simulink model "Filter_testaus_uusi"  (R2017b)
settings: Solver=FixedStepDiscrete  StartTime=0.0  StopTime=10  FixedStep=1/44100  RelTol=1e-3
(part 2 of 4)

== system Filter_testaus_uusi/Highpass/HighpassH/Resonator100 ==
  In1 : Inport
  Constant : Constant  Value=0i
  Delay : Delay  DelayLength=1
  Gain : Gain  Gain=-0.93539-0.3536i
  GainH : Gain  Gain=-0.16604+0.98612i
  Real-Imag to Complex : RealImagToComplex
  Sum1 : Sum  Inputs=|++
  Out1 : Outport
  wires:
  Constant/1 -> Real-Imag to Complex/2
  Real-Imag to Complex/1 -> Sum1/1
  In1/1 -> Real-Imag to Complex/1
  GainH/1 -> Out1/1
  Gain/1 -> Sum1/2
  Delay/1 -> Gain/1
  Sum1/1 -> Delay/1, GainH/1

== system Filter_testaus_uusi/Highpass/HighpassH/Resonator101 ==
  In1 : Inport
  Constant : Constant  Value=0i
  Delay : Delay  DelayLength=1
  Gain : Gain  Gain=-0.9252-0.37947i
  GainH : Gain  Gain=0.17973-0.98372i
  Real-Imag to Complex : RealImagToComplex
  Sum1 : Sum  Inputs=|++
  Out1 : Outport
  wires:
  Constant/1 -> Real-Imag to Complex/2
  Real-Imag to Complex/1 -> Sum1/1
  In1/1 -> Real-Imag to Complex/1
  GainH/1 -> Out1/1
  Gain/1 -> Sum1/2
  Delay/1 -> Gain/1
  Sum1/1 -> Delay/1, GainH/1

== system Filter_testaus_uusi/Highpass/HighpassH/Resonator102 ==
  In1 : Inport
  Constant : Constant  Value=0i
  Delay : Delay  DelayLength=1
  Gain : Gain  Gain=-0.9143-0.40504i
  GainH : Gain  Gain=-0.19339+0.98112i
  Real-Imag to Complex : RealImagToComplex
  Sum1 : Sum  Inputs=|++
  Out1 : Outport
  wires:
  Constant/1 -> Real-Imag to Complex/2
  Real-Imag to Complex/1 -> Sum1/1
  In1/1 -> Real-Imag to Complex/1
  GainH/1 -> Out1/1
  Gain/1 -> Sum1/2
  Delay/1 -> Gain/1
  Sum1/1 -> Delay/1, GainH/1

== system Filter_testaus_uusi/Highpass/HighpassH/Resonator103 ==
  In1 : Inport
  Constant : Constant  Value=0i
  Delay : Delay  DelayLength=1
  Gain : Gain  Gain=-0.90269-0.4303i
  GainH : Gain  Gain=0.20701-0.97834i
  Real-Imag to Complex : RealImagToComplex
  Sum1 : Sum  Inputs=|++
  Out1 : Outport
  wires:
  Constant/1 -> Real-Imag to Complex/2
  Real-Imag to Complex/1 -> Sum1/1
  In1/1 -> Real-Imag to Complex/1
  GainH/1 -> Out1/1
  Gain/1 -> Sum1/2
  Delay/1 -> Gain/1
  Sum1/1 -> Delay/1, GainH/1

== system Filter_testaus_uusi/Highpass/HighpassH/Resonator104 ==
  In1 : Inport
  Constant : Constant  Value=0i
  Delay : Delay  DelayLength=1
  Gain : Gain  Gain=-0.89037-0.45523i
  GainH : Gain  Gain=-0.22058+0.97537i
  Real-Imag to Complex : RealImagToComplex
  Sum1 : Sum  Inputs=|++
  Out1 : Outport
  wires:
  Constant/1 -> Real-Imag to Complex/2
  Real-Imag to Complex/1 -> Sum1/1
  In1/1 -> Real-Imag to Complex/1
  GainH/1 -> Out1/1
  Gain/1 -> Sum1/2
  Delay/1 -> Gain/1
  Sum1/1 -> Delay/1, GainH/1

== system Filter_testaus_uusi/Highpass/HighpassH/Resonator105 ==
  In1 : Inport
  Constant : Constant  Value=0i
  Delay : Delay  DelayLength=1
  Gain : Gain  Gain=-0.87738-0.4798i
  GainH : Gain  Gain=0.23412-0.97221i
  Real-Imag to Complex : RealImagToComplex
  Sum1 : Sum  Inputs=|++
  Out1 : Outport
  wires:
  Constant/1 -> Real-Imag to Complex/2
  Real-Imag to Complex/1 -> Sum1/1
  In1/1 -> Real-Imag to Complex/1
  GainH/1 -> Out1/1
  Gain/1 -> Sum1/2
  Delay/1 -> Gain/1
  Sum1/1 -> Delay/1, GainH/1

== system Filter_testaus_uusi/Highpass/HighpassH/Resonator106 ==
  In1 : Inport
  Constant : Constant  Value=0i
  Delay : Delay  DelayLength=1
  Gain : Gain  Gain=-0.8637-0.50401i
  GainH : Gain  Gain=-0.24761+0.96886i
  Real-Imag to Complex : RealImagToComplex
  Sum1 : Sum  Inputs=|++
  Out1 : Outport
  wires:
  Constant/1 -> Real-Imag to Complex/2
  Real-Imag to Complex/1 -> Sum1/1
  In1/1 -> Real-Imag to Complex/1
  GainH/1 -> Out1/1
  Gain/1 -> Sum1/2
  Delay/1 -> Gain/1
  Sum1/1 -> Delay/1, GainH/1

== system Filter_testaus_uusi/Highpass/HighpassH/Resonator107 ==
  In1 : Inport
  Constant : Constant  Value=0i
  Delay : Delay  DelayLength=1
  Gain : Gain  Gain=-0.84936-0.52782i
  GainH : Gain  Gain=0.26106-0.96532i
  Real-Imag to Complex : RealImagToComplex
  Sum1 : Sum  Inputs=|++
  Out1 : Outport
  wires:
  Constant/1 -> Real-Imag to Complex/2
  Real-Imag to Complex/1 -> Sum1/1
  In1/1 -> Real-Imag to Complex/1
  GainH/1 -> Out1/1
  Gain/1 -> Sum1/2
  Delay/1 -> Gain/1
  Sum1/1 -> Delay/1, GainH/1

== system Filter_testaus_uusi/Highpass/HighpassH/Resonator108 ==
  In1 : Inport
  Constant : Constant  Value=0i
  Delay : Delay  DelayLength=1
  Gain : Gain  Gain=-0.83435-0.55123i
  GainH : Gain  Gain=-0.27445+0.9616i
  Real-Imag to Complex : RealImagToComplex
  Sum1 : Sum  Inputs=|++
  Out1 : Outport
  wires:
  Constant/1 -> Real-Imag to Complex/2
  Real-Imag to Complex/1 -> Sum1/1
  In1/1 -> Real-Imag to Complex/1
  GainH/1 -> Out1/1
  Gain/1 -> Sum1/2
  Delay/1 -> Gain/1
  Sum1/1 -> Delay/1, GainH/1

== system Filter_testaus_uusi/Highpass/HighpassH/Resonator109 ==
  In1 : Inport
  Constant : Constant  Value=0i
  Delay : Delay  DelayLength=1
  Gain : Gain  Gain=-0.81871-0.57421i
  GainH : Gain  Gain=0.28779-0.95769i
  Real-Imag to Complex : RealImagToComplex
  Sum1 : Sum  Inputs=|++
  Out1 : Outport
  wires:
  Constant/1 -> Real-Imag to Complex/2
  Real-Imag to Complex/1 -> Sum1/1
  In1/1 -> Real-Imag to Complex/1
  GainH/1 -> Out1/1
  Gain/1 -> Sum1/2
  Delay/1 -> Gain/1
  Sum1/1 -> Delay/1, GainH/1

== system Filter_testaus_uusi/Highpass/HighpassH/Resonator11 ==
  In1 : Inport
  Constant : Constant  Value=0i
  Delay : Delay  DelayLength=1
  Gain : Gain  Gain=0.51596+0.85661i
  GainH : Gain  Gain=0.87738+0.4798i
  Real-Imag to Complex : RealImagToComplex
  Sum1 : Sum  Inputs=|++
  Out1 : Outport
  wires:
  Constant/1 -> Real-Imag to Complex/2
  Real-Imag to Complex/1 -> Sum1/1
  In1/1 -> Real-Imag to Complex/1
  GainH/1 -> Out1/1
  Gain/1 -> Sum1/2
  Delay/1 -> Gain/1
  Sum1/1 -> Delay/1, GainH/1

== system Filter_testaus_uusi/Highpass/HighpassH/Resonator110 ==
  In1 : Inport
  Constant : Constant  Value=0i
  Delay : Delay  DelayLength=1
  Gain : Gain  Gain=-0.80243-0.59675i
  GainH : Gain  Gain=-0.30107+0.9536i
  Real-Imag to Complex : RealImagToComplex
  Sum1 : Sum  Inputs=|++
  Out1 : Outport
  wires:
  Constant/1 -> Real-Imag to Complex/2
  Real-Imag to Complex/1 -> Sum1/1
  In1/1 -> Real-Imag to Complex/1
  GainH/1 -> Out1/1
  Gain/1 -> Sum1/2
  Delay/1 -> Gain/1
  Sum1/1 -> Delay/1, GainH/1

== system Filter_testaus_uusi/Highpass/HighpassH/Resonator111 ==
  In1 : Inport
  Constant : Constant  Value=0i
  Delay : Delay  DelayLength=1
  Gain : Gain  Gain=-0.78553-0.61882i
  GainH : Gain  Gain=0.3143-0.94932i
  Real-Imag to Complex : RealImagToComplex
  Sum1 : Sum  Inputs=|++
  Out1 : Outport
  wires:
  Constant/1 -> Real-Imag to Complex/2
  Real-Imag to Complex/1 -> Sum1/1
  In1/1 -> Real-Imag to Complex/1
  GainH/1 -> Out1/1
  Gain/1 -> Sum1/2
  Delay/1 -> Gain/1
  Sum1/1 -> Delay/1, GainH/1

== system Filter_testaus_uusi/Highpass/HighpassH/Resonator112 ==
  In1 : Inport
  Constant : Constant  Value=0i
  Delay : Delay  DelayLength=1
  Gain : Gain  Gain=-0.76803-0.64042i
  GainH : Gain  Gain=-0.32747+0.94486i
  Real-Imag to Complex : RealImagToComplex
  Sum1 : Sum  Inputs=|++
  Out1 : Outport
  wires:
  Constant/1 -> Real-Imag to Complex/2
  Real-Imag to Complex/1 -> Sum1/1
  In1/1 -> Real-Imag to Complex/1
  GainH/1 -> Out1/1
  Gain/1 -> Sum1/2
  Delay/1 -> Gain/1
  Sum1/1 -> Delay/1, GainH/1

== system Filter_testaus_uusi/Highpass/HighpassH/Resonator113 ==
  In1 : Inport
  Constant : Constant  Value=0i
  Delay : Delay  DelayLength=1
  Gain : Gain  Gain=-0.74993-0.66152i
  GainH : Gain  Gain=0.34057-0.94022i
  Real-Imag to Complex : RealImagToComplex
  Sum1 : Sum  Inputs=|++
  Out1 : Outport
  wires:
  Constant/1 -> Real-Imag to Complex/2
  Real-Imag to Complex/1 -> Sum1/1
  In1/1 -> Real-Imag to Complex/1
  GainH/1 -> Out1/1
  Gain/1 -> Sum1/2
  Delay/1 -> Gain/1
  Sum1/1 -> Delay/1, GainH/1

== system Filter_testaus_uusi/Highpass/HighpassH/Resonator114 ==
  In1 : Inport
  Constant : Constant  Value=0i
  Delay : Delay  DelayLength=1
  Gain : Gain  Gain=-0.73125-0.68211i
  GainH : Gain  Gain=-0.3536+0.93539i
  Real-Imag to Complex : RealImagToComplex
  Sum1 : Sum  Inputs=|++
  Out1 : Outport
  wires:
  Constant/1 -> Real-Imag to Complex/2
  Real-Imag to Complex/1 -> Sum1/1
  In1/1 -> Real-Imag to Complex/1
  GainH/1 -> Out1/1
  Gain/1 -> Sum1/2
  Delay/1 -> Gain/1
  Sum1/1 -> Delay/1, GainH/1

== system Filter_testaus_uusi/Highpass/HighpassH/Resonator115 ==
  In1 : Inport
  Constant : Constant  Value=0i
  Delay : Delay  DelayLength=1
  Gain : Gain  Gain=-0.712-0.70218i
  GainH : Gain  Gain=0.36657-0.93039i
  Real-Imag to Complex : RealImagToComplex
  Sum1 : Sum  Inputs=|++
  Out1 : Outport
  wires:
  Constant/1 -> Real-Imag to Complex/2
  Real-Imag to Complex/1 -> Sum1/1
  In1/1 -> Real-Imag to Complex/1
  GainH/1 -> Out1/1
  Gain/1 -> Sum1/2
  Delay/1 -> Gain/1
  Sum1/1 -> Delay/1, GainH/1

== system Filter_testaus_uusi/Highpass/HighpassH/Resonator116 ==
  In1 : Inport
  Constant : Constant  Value=0i
  Delay : Delay  DelayLength=1
  Gain : Gain  Gain=-0.69221-0.7217i
  GainH : Gain  Gain=-0.37947+0.9252i
  Real-Imag to Complex : RealImagToComplex
  Sum1 : Sum  Inputs=|++
  Out1 : Outport
  wires:
  Constant/1 -> Real-Imag to Complex/2
  Real-Imag to Complex/1 -> Sum1/1
  In1/1 -> Real-Imag to Complex/1
  GainH/1 -> Out1/1
  Gain/1 -> Sum1/2
  Delay/1 -> Gain/1
  Sum1/1 -> Delay/1, GainH/1

== system Filter_testaus_uusi/Highpass/HighpassH/Resonator117 ==
  In1 : Inport
  Constant : Constant  Value=0i
  Delay : Delay  DelayLength=1
  Gain : Gain  Gain=-0.67188-0.74066i
  GainH : Gain  Gain=0.39229-0.91984i
  Real-Imag to Complex : RealImagToComplex
  Sum1 : Sum  Inputs=|++
  Out1 : Outport
  wires:
  Constant/1 -> Real-Imag to Complex/2
  Real-Imag to Complex/1 -> Sum1/1
  In1/1 -> Real-Imag to Complex/1
  GainH/1 -> Out1/1
  Gain/1 -> Sum1/2
  Delay/1 -> Gain/1
  Sum1/1 -> Delay/1, GainH/1

== system Filter_testaus_uusi/Highpass/HighpassH/Resonator118 ==
  In1 : Inport
  Constant : Constant  Value=0i
  Delay : Delay  DelayLength=1
  Gain : Gain  Gain=-0.65103-0.75905i
  GainH : Gain  Gain=-0.40504+0.9143i
  Real-Imag to Complex : RealImagToComplex
  Sum1 : Sum  Inputs=|++
  Out1 : Outport
  wires:
  Constant/1 -> Real-Imag to Complex/2
  Real-Imag to Complex/1 -> Sum1/1
  In1/1 -> Real-Imag to Complex/1
  GainH/1 -> Out1/1
  Gain/1 -> Sum1/2
  Delay/1 -> Gain/1
  Sum1/1 -> Delay/1, GainH/1

== system Filter_testaus_uusi/Highpass/HighpassH/Resonator119 ==
  In1 : Inport
  Constant : Constant  Value=0i
  Delay : Delay  DelayLength=1
  Gain : Gain  Gain=-0.62968-0.77685i
  GainH : Gain  Gain=0.41771-0.90858i
  Real-Imag to Complex : RealImagToComplex
  Sum1 : Sum  Inputs=|++
  Out1 : Outport
  wires:
  Constant/1 -> Real-Imag to Complex/2
  Real-Imag to Complex/1 -> Sum1/1
  In1/1 -> Real-Imag to Complex/1
  GainH/1 -> Out1/1
  Gain/1 -> Sum1/2
  Delay/1 -> Gain/1
  Sum1/1 -> Delay/1, GainH/1

== system Filter_testaus_uusi/Highpass/HighpassH/Resonator12 ==
  In1 : Inport
  Constant : Constant  Value=0i
  Delay : Delay  DelayLength=1
  Gain : Gain  Gain=0.49195+0.87062i
  GainH : Gain  Gain=-0.87062-0.49195i
  Real-Imag to Complex : RealImagToComplex
  Sum1 : Sum  Inputs=|++
  Out1 : Outport
  wires:
  Constant/1 -> Real-Imag to Complex/2
  Real-Imag to Complex/1 -> Sum1/1
  In1/1 -> Real-Imag to Complex/1
  GainH/1 -> Out1/1
  Gain/1 -> Sum1/2
  Delay/1 -> Gain/1
  Sum1/1 -> Delay/1, GainH/1

== system Filter_testaus_uusi/Highpass/HighpassH/Resonator120 ==
  In1 : Inport
  Constant : Constant  Value=0i
  Delay : Delay  DelayLength=1
  Gain : Gain  Gain=-0.60784-0.79406i
  GainH : Gain  Gain=-0.4303+0.90269i
  Real-Imag to Complex : RealImagToComplex
  Sum1 : Sum  Inputs=|++
  Out1 : Outport
  wires:
  Constant/1 -> Real-Imag to Complex/2
  Real-Imag to Complex/1 -> Sum1/1
  In1/1 -> Real-Imag to Complex/1
  GainH/1 -> Out1/1
  Gain/1 -> Sum1/2
  Delay/1 -> Gain/1
  Sum1/1 -> Delay/1, GainH/1

== system Filter_testaus_uusi/Highpass/HighpassH/Resonator121 ==
  In1 : Inport
  Constant : Constant  Value=0i
  Delay : Delay  DelayLength=1
  Gain : Gain  Gain=-0.58553-0.81065i
  GainH : Gain  Gain=0.44281-0.89662i
  Real-Imag to Complex : RealImagToComplex
  Sum1 : Sum  Inputs=|++
  Out1 : Outport
  wires:
  Constant/1 -> Real-Imag to Complex/2
  Real-Imag to Complex/1 -> Sum1/1
  In1/1 -> Real-Imag to Complex/1
  GainH/1 -> Out1/1
  Gain/1 -> Sum1/2
  Delay/1 -> Gain/1
  Sum1/1 -> Delay/1, GainH/1

== system Filter_testaus_uusi/Highpass/HighpassH/Resonator122 ==
  In1 : Inport
  Constant : Constant  Value=0i
  Delay : Delay  DelayLength=1
  Gain : Gain  Gain=-0.56277-0.82661i
  GainH : Gain  Gain=-0.45523+0.89037i
  Real-Imag to Complex : RealImagToComplex
  Sum1 : Sum  Inputs=|++
  Out1 : Outport
  wires:
  Constant/1 -> Real-Imag to Complex/2
  Real-Imag to Complex/1 -> Sum1/1
  In1/1 -> Real-Imag to Complex/1
  GainH/1 -> Out1/1
  Gain/1 -> Sum1/2
  Delay/1 -> Gain/1
  Sum1/1 -> Delay/1, GainH/1

== system Filter_testaus_uusi/Highpass/HighpassH/Resonator123 ==
  In1 : Inport
  Constant : Constant  Value=0i
  Delay : Delay  DelayLength=1
  Gain : Gain  Gain=-0.53958-0.84194i
  GainH : Gain  Gain=0.46756-0.88396i
  Real-Imag to Complex : RealImagToComplex
  Sum1 : Sum  Inputs=|++
  Out1 : Outport
  wires:
  Constant/1 -> Real-Imag to Complex/2
  Real-Imag to Complex/1 -> Sum1/1
  In1/1 -> Real-Imag to Complex/1
  GainH/1 -> Out1/1
  Gain/1 -> Sum1/2
  Delay/1 -> Gain/1
  Sum1/1 -> Delay/1, GainH/1

== system Filter_testaus_uusi/Highpass/HighpassH/Resonator124 ==
  In1 : Inport
  Constant : Constant  Value=0i
  Delay : Delay  DelayLength=1
  Gain : Gain  Gain=-0.51596-0.85661i
  GainH : Gain  Gain=-0.4798+0.87738i
  Real-Imag to Complex : RealImagToComplex
  Sum1 : Sum  Inputs=|++
  Out1 : Outport
  wires:
  Constant/1 -> Real-Imag to Complex/2
  Real-Imag to Complex/1 -> Sum1/1
  In1/1 -> Real-Imag to Complex/1
  GainH/1 -> Out1/1
  Gain/1 -> Sum1/2
  Delay/1 -> Gain/1
  Sum1/1 -> Delay/1, GainH/1

== system Filter_testaus_uusi/Highpass/HighpassH/Resonator125 ==
  In1 : Inport
  Constant : Constant  Value=0i
  Delay : Delay  DelayLength=1
  Gain : Gain  Gain=-0.49195-0.87062i
  GainH : Gain  Gain=0.49195-0.87062i
  Real-Imag to Complex : RealImagToComplex
  Sum1 : Sum  Inputs=|++
  Out1 : Outport
  wires:
  Constant/1 -> Real-Imag to Complex/2
  Real-Imag to Complex/1 -> Sum1/1
  In1/1 -> Real-Imag to Complex/1
  GainH/1 -> Out1/1
  Gain/1 -> Sum1/2
  Delay/1 -> Gain/1
  Sum1/1 -> Delay/1, GainH/1

== system Filter_testaus_uusi/Highpass/HighpassH/Resonator126 ==
  In1 : Inport
  Constant : Constant  Value=0i
  Delay : Delay  DelayLength=1
  Gain : Gain  Gain=-0.46756-0.88396i
  GainH : Gain  Gain=-0.50401+0.8637i
  Real-Imag to Complex : RealImagToComplex
  Sum1 : Sum  Inputs=|++
  Out1 : Outport
  wires:
  Constant/1 -> Real-Imag to Complex/2
  Real-Imag to Complex/1 -> Sum1/1
  In1/1 -> Real-Imag to Complex/1
  GainH/1 -> Out1/1
  Gain/1 -> Sum1/2
  Delay/1 -> Gain/1
  Sum1/1 -> Delay/1, GainH/1

== system Filter_testaus_uusi/Highpass/HighpassH/Resonator127 ==
  In1 : Inport
  Constant : Constant  Value=0i
  Delay : Delay  DelayLength=1
  Gain : Gain  Gain=-0.44281-0.89662i
  GainH : Gain  Gain=0.51596-0.85661i
  Real-Imag to Complex : RealImagToComplex
  Sum1 : Sum  Inputs=|++
  Out1 : Outport
  wires:
  Constant/1 -> Real-Imag to Complex/2
  Real-Imag to Complex/1 -> Sum1/1
  In1/1 -> Real-Imag to Complex/1
  GainH/1 -> Out1/1
  Gain/1 -> Sum1/2
  Delay/1 -> Gain/1
  Sum1/1 -> Delay/1, GainH/1

== system Filter_testaus_uusi/Highpass/HighpassH/Resonator128 ==
  In1 : Inport
  Constant : Constant  Value=0i
  Delay : Delay  DelayLength=1
  Gain : Gain  Gain=-0.41771-0.90858i
  GainH : Gain  Gain=-0.52782+0.84936i
  Real-Imag to Complex : RealImagToComplex
  Sum1 : Sum  Inputs=|++
  Out1 : Outport
  wires:
  Constant/1 -> Real-Imag to Complex/2
  Real-Imag to Complex/1 -> Sum1/1
  In1/1 -> Real-Imag to Complex/1
  GainH/1 -> Out1/1
  Gain/1 -> Sum1/2
  Delay/1 -> Gain/1
  Sum1/1 -> Delay/1, GainH/1

== system Filter_testaus_uusi/Highpass/HighpassH/Resonator129 ==
  In1 : Inport
  Constant : Constant  Value=0i
  Delay : Delay  DelayLength=1
  Gain : Gain  Gain=-0.39229-0.91984i
  GainH : Gain  Gain=0.53958-0.84194i
  Real-Imag to Complex : RealImagToComplex
  Sum1 : Sum  Inputs=|++
  Out1 : Outport
  wires:
  Constant/1 -> Real-Imag to Complex/2
  Real-Imag to Complex/1 -> Sum1/1
  In1/1 -> Real-Imag to Complex/1
  GainH/1 -> Out1/1
  Gain/1 -> Sum1/2
  Delay/1 -> Gain/1
  Sum1/1 -> Delay/1, GainH/1

== system Filter_testaus_uusi/Highpass/HighpassH/Resonator13 ==
  In1 : Inport
  Constant : Constant  Value=0i
  Delay : Delay  DelayLength=1
  Gain : Gain  Gain=0.46756+0.88396i
  GainH : Gain  Gain=0.8637+0.50401i
  Real-Imag to Complex : RealImagToComplex
  Sum1 : Sum  Inputs=|++
  Out1 : Outport
  wires:
  Constant/1 -> Real-Imag to Complex/2
  Real-Imag to Complex/1 -> Sum1/1
  In1/1 -> Real-Imag to Complex/1
  GainH/1 -> Out1/1
  Gain/1 -> Sum1/2
  Delay/1 -> Gain/1
  Sum1/1 -> Delay/1, GainH/1

== system Filter_testaus_uusi/Highpass/HighpassH/Resonator130 ==
  In1 : Inport
  Constant : Constant  Value=0i
  Delay : Delay  DelayLength=1
  Gain : Gain  Gain=-0.36657-0.93039i
  GainH : Gain  Gain=-0.55123+0.83435i
  Real-Imag to Complex : RealImagToComplex
  Sum1 : Sum  Inputs=|++
  Out1 : Outport
  wires:
  Constant/1 -> Real-Imag to Complex/2
  Real-Imag to Complex/1 -> Sum1/1
  In1/1 -> Real-Imag to Complex/1
  GainH/1 -> Out1/1
  Gain/1 -> Sum1/2
  Delay/1 -> Gain/1
  Sum1/1 -> Delay/1, GainH/1

== system Filter_testaus_uusi/Highpass/HighpassH/Resonator131 ==
  In1 : Inport
  Constant : Constant  Value=0i
  Delay : Delay  DelayLength=1
  Gain : Gain  Gain=-0.34057-0.94022i
  GainH : Gain  Gain=0.56277-0.82661i
  Real-Imag to Complex : RealImagToComplex
  Sum1 : Sum  Inputs=|++
  Out1 : Outport
  wires:
  Constant/1 -> Real-Imag to Complex/2
  Real-Imag to Complex/1 -> Sum1/1
  In1/1 -> Real-Imag to Complex/1
  GainH/1 -> Out1/1
  Gain/1 -> Sum1/2
  Delay/1 -> Gain/1
  Sum1/1 -> Delay/1, GainH/1

== system Filter_testaus_uusi/Highpass/HighpassH/Resonator132 ==
  In1 : Inport
  Constant : Constant  Value=0i
  Delay : Delay  DelayLength=1
  Gain : Gain  Gain=-0.3143-0.94932i
  GainH : Gain  Gain=-0.57421+0.81871i
  Real-Imag to Complex : RealImagToComplex
  Sum1 : Sum  Inputs=|++
  Out1 : Outport
  wires:
  Constant/1 -> Real-Imag to Complex/2
  Real-Imag to Complex/1 -> Sum1/1
  In1/1 -> Real-Imag to Complex/1
  GainH/1 -> Out1/1
  Gain/1 -> Sum1/2
  Delay/1 -> Gain/1
  Sum1/1 -> Delay/1, GainH/1

== system Filter_testaus_uusi/Highpass/HighpassH/Resonator133 ==
  In1 : Inport
  Constant : Constant  Value=0i
  Delay : Delay  DelayLength=1
  Gain : Gain  Gain=-0.28779-0.95769i
  GainH : Gain  Gain=0.58553-0.81065i
  Real-Imag to Complex : RealImagToComplex
  Sum1 : Sum  Inputs=|++
  Out1 : Outport
  wires:
  Constant/1 -> Real-Imag to Complex/2
  Real-Imag to Complex/1 -> Sum1/1
  In1/1 -> Real-Imag to Complex/1
  GainH/1 -> Out1/1
  Gain/1 -> Sum1/2
  Delay/1 -> Gain/1
  Sum1/1 -> Delay/1, GainH/1

== system Filter_testaus_uusi/Highpass/HighpassH/Resonator134 ==
  In1 : Inport
  Constant : Constant  Value=0i
  Delay : Delay  DelayLength=1
  Gain : Gain  Gain=-0.26106-0.96532i
  GainH : Gain  Gain=-0.59675+0.80243i
  Real-Imag to Complex : RealImagToComplex
  Sum1 : Sum  Inputs=|++
  Out1 : Outport
  wires:
  Constant/1 -> Real-Imag to Complex/2
  Real-Imag to Complex/1 -> Sum1/1
  In1/1 -> Real-Imag to Complex/1
  GainH/1 -> Out1/1
  Gain/1 -> Sum1/2
  Delay/1 -> Gain/1
  Sum1/1 -> Delay/1, GainH/1

== system Filter_testaus_uusi/Highpass/HighpassH/Resonator135 ==
  In1 : Inport
  Constant : Constant  Value=0i
  Delay : Delay  DelayLength=1
  Gain : Gain  Gain=-0.23412-0.97221i
  GainH : Gain  Gain=0.60784-0.79406i
  Real-Imag to Complex : RealImagToComplex
  Sum1 : Sum  Inputs=|++
  Out1 : Outport
  wires:
  Constant/1 -> Real-Imag to Complex/2
  Real-Imag to Complex/1 -> Sum1/1
  In1/1 -> Real-Imag to Complex/1
  GainH/1 -> Out1/1
  Gain/1 -> Sum1/2
  Delay/1 -> Gain/1
  Sum1/1 -> Delay/1, GainH/1

== system Filter_testaus_uusi/Highpass/HighpassH/Resonator136 ==
  In1 : Inport
  Constant : Constant  Value=0i
  Delay : Delay  DelayLength=1
  Gain : Gain  Gain=-0.20701-0.97834i
  GainH : Gain  Gain=-0.61882+0.78553i
  Real-Imag to Complex : RealImagToComplex
  Sum1 : Sum  Inputs=|++
  Out1 : Outport
  wires:
  Constant/1 -> Real-Imag to Complex/2
  Real-Imag to Complex/1 -> Sum1/1
  In1/1 -> Real-Imag to Complex/1
  GainH/1 -> Out1/1
  Gain/1 -> Sum1/2
  Delay/1 -> Gain/1
  Sum1/1 -> Delay/1, GainH/1

== system Filter_testaus_uusi/Highpass/HighpassH/Resonator137 ==
  In1 : Inport
  Constant : Constant  Value=0i
  Delay : Delay  DelayLength=1
  Gain : Gain  Gain=-0.17973-0.98372i
  GainH : Gain  Gain=0.62968-0.77685i
  Real-Imag to Complex : RealImagToComplex
  Sum1 : Sum  Inputs=|++
  Out1 : Outport
  wires:
  Constant/1 -> Real-Imag to Complex/2
  Real-Imag to Complex/1 -> Sum1/1
  In1/1 -> Real-Imag to Complex/1
  GainH/1 -> Out1/1
  Gain/1 -> Sum1/2
  Delay/1 -> Gain/1
  Sum1/1 -> Delay/1, GainH/1

== system Filter_testaus_uusi/Highpass/HighpassH/Resonator138 ==
  In1 : Inport
  Constant : Constant  Value=0i
  Delay : Delay  DelayLength=1
  Gain : Gain  Gain=-0.15231-0.98833i
  GainH : Gain  Gain=-0.64042+0.76803i
  Real-Imag to Complex : RealImagToComplex
  Sum1 : Sum  Inputs=|++
  Out1 : Outport
  wires:
  Constant/1 -> Real-Imag to Complex/2
  Real-Imag to Complex/1 -> Sum1/1
  In1/1 -> Real-Imag to Complex/1
  GainH/1 -> Out1/1
  Gain/1 -> Sum1/2
  Delay/1 -> Gain/1
  Sum1/1 -> Delay/1, GainH/1

== system Filter_testaus_uusi/Highpass/HighpassH/Resonator139 ==
  In1 : Inport
  Constant : Constant  Value=0i
  Delay : Delay  DelayLength=1
  Gain : Gain  Gain=-0.12478-0.99218i
  GainH : Gain  Gain=0.65103-0.75905i
  Real-Imag to Complex : RealImagToComplex
  Sum1 : Sum  Inputs=|++
  Out1 : Outport
  wires:
  Constant/1 -> Real-Imag to Complex/2
  Real-Imag to Complex/1 -> Sum1/1
  In1/1 -> Real-Imag to Complex/1
  GainH/1 -> Out1/1
  Gain/1 -> Sum1/2
  Delay/1 -> Gain/1
  Sum1/1 -> Delay/1, GainH/1

== system Filter_testaus_uusi/Highpass/HighpassH/Resonator14 ==
  In1 : Inport
  Constant : Constant  Value=0i
  Delay : Delay  DelayLength=1
  Gain : Gain  Gain=0.44281+0.89662i
  GainH : Gain  Gain=-0.85661-0.51596i
  Real-Imag to Complex : RealImagToComplex
  Sum1 : Sum  Inputs=|++
  Out1 : Outport
  wires:
  Constant/1 -> Real-Imag to Complex/2
  Real-Imag to Complex/1 -> Sum1/1
  In1/1 -> Real-Imag to Complex/1
  GainH/1 -> Out1/1
  Gain/1 -> Sum1/2
  Delay/1 -> Gain/1
  Sum1/1 -> Delay/1, GainH/1

== system Filter_testaus_uusi/Highpass/HighpassH/Resonator140 ==
  In1 : Inport
  Constant : Constant  Value=0i
  Delay : Delay  DelayLength=1
  Gain : Gain  Gain=-0.097152-0.99527i
  GainH : Gain  Gain=-0.66152+0.74993i
  Real-Imag to Complex : RealImagToComplex
  Sum1 : Sum  Inputs=|++
  Out1 : Outport
  wires:
  Constant/1 -> Real-Imag to Complex/2
  Real-Imag to Complex/1 -> Sum1/1
  In1/1 -> Real-Imag to Complex/1
  GainH/1 -> Out1/1
  Gain/1 -> Sum1/2
  Delay/1 -> Gain/1
  Sum1/1 -> Delay/1, GainH/1

== system Filter_testaus_uusi/Highpass/HighpassH/Resonator141 ==
  In1 : Inport
  Constant : Constant  Value=0i
  Delay : Delay  DelayLength=1
  Gain : Gain  Gain=-0.069448-0.99759i
  GainH : Gain  Gain=0.67188-0.74066i
  Real-Imag to Complex : RealImagToComplex
  Sum1 : Sum  Inputs=|++
  Out1 : Outport
  wires:
  Constant/1 -> Real-Imag to Complex/2
  Real-Imag to Complex/1 -> Sum1/1
  In1/1 -> Real-Imag to Complex/1
  GainH/1 -> Out1/1
  Gain/1 -> Sum1/2
  Delay/1 -> Gain/1
  Sum1/1 -> Delay/1, GainH/1

== system Filter_testaus_uusi/Highpass/HighpassH/Resonator142 ==
  In1 : Inport
  Constant : Constant  Value=0i
  Delay : Delay  DelayLength=1
  Gain : Gain  Gain=-0.04169-0.99913i
  GainH : Gain  Gain=-0.68211+0.73125i
  Real-Imag to Complex : RealImagToComplex
  Sum1 : Sum  Inputs=|++
  Out1 : Outport
  wires:
  Constant/1 -> Real-Imag to Complex/2
  Real-Imag to Complex/1 -> Sum1/1
  In1/1 -> Real-Imag to Complex/1
  GainH/1 -> Out1/1
  Gain/1 -> Sum1/2
  Delay/1 -> Gain/1
  Sum1/1 -> Delay/1, GainH/1

== system Filter_testaus_uusi/Highpass/HighpassH/Resonator143 ==
  In1 : Inport
  Constant : Constant  Value=0i
  Delay : Delay  DelayLength=1
  Gain : Gain  Gain=-0.0139-0.9999i
  GainH : Gain  Gain=0.69221-0.7217i
  Real-Imag to Complex : RealImagToComplex
  Sum1 : Sum  Inputs=|++
  Out1 : Outport
  wires:
  Constant/1 -> Real-Imag to Complex/2
  Real-Imag to Complex/1 -> Sum1/1
  In1/1 -> Real-Imag to Complex/1
  GainH/1 -> Out1/1
  Gain/1 -> Sum1/2
  Delay/1 -> Gain/1
  Sum1/1 -> Delay/1, GainH/1

== system Filter_testaus_uusi/Highpass/HighpassH/Resonator144 ==
  In1 : Inport
  Constant : Constant  Value=0i
  Delay : Delay  DelayLength=1
  Gain : Gain  Gain=0.0139-0.9999i
  GainH : Gain  Gain=-0.70218+0.712i
  Real-Imag to Complex : RealImagToComplex
  Sum1 : Sum  Inputs=|++
  Out1 : Outport
  wires:
  Constant/1 -> Real-Imag to Complex/2
  Real-Imag to Complex/1 -> Sum1/1
  In1/1 -> Real-Imag to Complex/1
  GainH/1 -> Out1/1
  Gain/1 -> Sum1/2
  Delay/1 -> Gain/1
  Sum1/1 -> Delay/1, GainH/1

== system Filter_testaus_uusi/Highpass/HighpassH/Resonator145 ==
  In1 : Inport
  Constant : Constant  Value=0i
  Delay : Delay  DelayLength=1
  Gain : Gain  Gain=0.04169-0.99913i
  GainH : Gain  Gain=0.712-0.70218i
  Real-Imag to Complex : RealImagToComplex
  Sum1 : Sum  Inputs=|++
  Out1 : Outport
  wires:
  Constant/1 -> Real-Imag to Complex/2
  Real-Imag to Complex/1 -> Sum1/1
  In1/1 -> Real-Imag to Complex/1
  GainH/1 -> Out1/1
  Gain/1 -> Sum1/2
  Delay/1 -> Gain/1
  Sum1/1 -> Delay/1, GainH/1

== system Filter_testaus_uusi/Highpass/HighpassH/Resonator146 ==
  In1 : Inport
  Constant : Constant  Value=0i
  Delay : Delay  DelayLength=1
  Gain : Gain  Gain=0.069448-0.99759i
  GainH : Gain  Gain=-0.7217+0.69221i
  Real-Imag to Complex : RealImagToComplex
  Sum1 : Sum  Inputs=|++
  Out1 : Outport
  wires:
  Constant/1 -> Real-Imag to Complex/2
  Real-Imag to Complex/1 -> Sum1/1
  In1/1 -> Real-Imag to Complex/1
  GainH/1 -> Out1/1
  Gain/1 -> Sum1/2
  Delay/1 -> Gain/1
  Sum1/1 -> Delay/1, GainH/1

== system Filter_testaus_uusi/Highpass/HighpassH/Resonator147 ==
  In1 : Inport
  Constant : Constant  Value=0i
  Delay : Delay  DelayLength=1
  Gain : Gain  Gain=0.097152-0.99527i
  GainH : Gain  Gain=0.73125-0.68211i
  Real-Imag to Complex : RealImagToComplex
  Sum1 : Sum  Inputs=|++
  Out1 : Outport
  wires:
  Constant/1 -> Real-Imag to Complex/2
  Real-Imag to Complex/1 -> Sum1/1
  In1/1 -> Real-Imag to Complex/1
  GainH/1 -> Out1/1
  Gain/1 -> Sum1/2
  Delay/1 -> Gain/1
  Sum1/1 -> Delay/1, GainH/1

== system Filter_testaus_uusi/Highpass/HighpassH/Resonator148 ==
  In1 : Inport
  Constant : Constant  Value=0i
  Delay : Delay  DelayLength=1
  Gain : Gain  Gain=0.12478-0.99218i
  GainH : Gain  Gain=-0.74066+0.67188i
  Real-Imag to Complex : RealImagToComplex
  Sum1 : Sum  Inputs=|++
  Out1 : Outport
  wires:
  Constant/1 -> Real-Imag to Complex/2
  Real-Imag to Complex/1 -> Sum1/1
  In1/1 -> Real-Imag to Complex/1
  GainH/1 -> Out1/1
  Gain/1 -> Sum1/2
  Delay/1 -> Gain/1
  Sum1/1 -> Delay/1, GainH/1

== system Filter_testaus_uusi/Highpass/HighpassH/Resonator149 ==
  In1 : Inport
  Constant : Constant  Value=0i
  Delay : Delay  DelayLength=1
  Gain : Gain  Gain=0.15231-0.98833i
  GainH : Gain  Gain=0.74993-0.66152i
  Real-Imag to Complex : RealImagToComplex
  Sum1 : Sum  Inputs=|++
  Out1 : Outport
  wires:
  Constant/1 -> Real-Imag to Complex/2
  Real-Imag to Complex/1 -> Sum1/1
  In1/1 -> Real-Imag to Complex/1
  GainH/1 -> Out1/1
  Gain/1 -> Sum1/2
  Delay/1 -> Gain/1
  Sum1/1 -> Delay/1, GainH/1

== system Filter_testaus_uusi/Highpass/HighpassH/Resonator15 ==
  In1 : Inport
  Constant : Constant  Value=0i
  Delay : Delay  DelayLength=1
  Gain : Gain  Gain=0.41771+0.90858i
  GainH : Gain  Gain=0.84936+0.52782i
  Real-Imag to Complex : RealImagToComplex
  Sum1 : Sum  Inputs=|++
  Out1 : Outport
  wires:
  Constant/1 -> Real-Imag to Complex/2
  Real-Imag to Complex/1 -> Sum1/1
  In1/1 -> Real-Imag to Complex/1
  GainH/1 -> Out1/1
  Gain/1 -> Sum1/2
  Delay/1 -> Gain/1
  Sum1/1 -> Delay/1, GainH/1

== system Filter_testaus_uusi/Highpass/HighpassH/Resonator150 ==
  In1 : Inport
  Constant : Constant  Value=0i
  Delay : Delay  DelayLength=1
  Gain : Gain  Gain=0.17973-0.98372i
  GainH : Gain  Gain=-0.75905+0.65103i
  Real-Imag to Complex : RealImagToComplex
  Sum1 : Sum  Inputs=|++
  Out1 : Outport
  wires:
  Constant/1 -> Real-Imag to Complex/2
  Real-Imag to Complex/1 -> Sum1/1
  In1/1 -> Real-Imag to Complex/1
  GainH/1 -> Out1/1
  Gain/1 -> Sum1/2
  Delay/1 -> Gain/1
  Sum1/1 -> Delay/1, GainH/1

== system Filter_testaus_uusi/Highpass/HighpassH/Resonator151 ==
  In1 : Inport
  Constant : Constant  Value=0i
  Delay : Delay  DelayLength=1
  Gain : Gain  Gain=0.20701-0.97834i
  GainH : Gain  Gain=0.76803-0.64042i
  Real-Imag to Complex : RealImagToComplex
  Sum1 : Sum  Inputs=|++
  Out1 : Outport
  wires:
  Constant/1 -> Real-Imag to Complex/2
  Real-Imag to Complex/1 -> Sum1/1
  In1/1 -> Real-Imag to Complex/1
  GainH/1 -> Out1/1
  Gain/1 -> Sum1/2
  Delay/1 -> Gain/1
  Sum1/1 -> Delay/1, GainH/1

== system Filter_testaus_uusi/Highpass/HighpassH/Resonator152 ==
  In1 : Inport
  Constant : Constant  Value=0i
  Delay : Delay  DelayLength=1
  Gain : Gain  Gain=0.23412-0.97221i
  GainH : Gain  Gain=-0.77685+0.62968i
  Real-Imag to Complex : RealImagToComplex
  Sum1 : Sum  Inputs=|++
  Out1 : Outport
  wires:
  Constant/1 -> Real-Imag to Complex/2
  Real-Imag to Complex/1 -> Sum1/1
  In1/1 -> Real-Imag to Complex/1
  GainH/1 -> Out1/1
  Gain/1 -> Sum1/2
  Delay/1 -> Gain/1
  Sum1/1 -> Delay/1, GainH/1

== system Filter_testaus_uusi/Highpass/HighpassH/Resonator153 ==
  In1 : Inport
  Constant : Constant  Value=0i
  Delay : Delay  DelayLength=1
  Gain : Gain  Gain=0.26106-0.96532i
  GainH : Gain  Gain=0.78553-0.61882i
  Real-Imag to Complex : RealImagToComplex
  Sum1 : Sum  Inputs=|++
  Out1 : Outport
  wires:
  Constant/1 -> Real-Imag to Complex/2
  Real-Imag to Complex/1 -> Sum1/1
  In1/1 -> Real-Imag to Complex/1
  GainH/1 -> Out1/1
  Gain/1 -> Sum1/2
  Delay/1 -> Gain/1
  Sum1/1 -> Delay/1, GainH/1

== system Filter_testaus_uusi/Highpass/HighpassH/Resonator154 ==
  In1 : Inport
  Constant : Constant  Value=0i
  Delay : Delay  DelayLength=1
  Gain : Gain  Gain=0.28779-0.95769i
  GainH : Gain  Gain=-0.79406+0.60784i
  Real-Imag to Complex : RealImagToComplex
  Sum1 : Sum  Inputs=|++
  Out1 : Outport
  wires:
  Constant/1 -> Real-Imag to Complex/2
  Real-Imag to Complex/1 -> Sum1/1
  In1/1 -> Real-Imag to Complex/1
  GainH/1 -> Out1/1
  Gain/1 -> Sum1/2
  Delay/1 -> Gain/1
  Sum1/1 -> Delay/1, GainH/1

== system Filter_testaus_uusi/Highpass/HighpassH/Resonator155 ==
  In1 : Inport
  Constant : Constant  Value=0i
  Delay : Delay  DelayLength=1
  Gain : Gain  Gain=0.3143-0.94932i
  GainH : Gain  Gain=0.80243-0.59675i
  Real-Imag to Complex : RealImagToComplex
  Sum1 : Sum  Inputs=|++
  Out1 : Outport
  wires:
  Constant/1 -> Real-Imag to Complex/2
  Real-Imag to Complex/1 -> Sum1/1
  In1/1 -> Real-Imag to Complex/1
  GainH/1 -> Out1/1
  Gain/1 -> Sum1/2
  Delay/1 -> Gain/1
  Sum1/1 -> Delay/1, GainH/1

== system Filter_testaus_uusi/Highpass/HighpassH/Resonator156 ==
  In1 : Inport
  Constant : Constant  Value=0i
  Delay : Delay  DelayLength=1
  Gain : Gain  Gain=0.34057-0.94022i
  GainH : Gain  Gain=-0.81065+0.58553i
  Real-Imag to Complex : RealImagToComplex
  Sum1 : Sum  Inputs=|++
  Out1 : Outport
  wires:
  Constant/1 -> Real-Imag to Complex/2
  Real-Imag to Complex/1 -> Sum1/1
  In1/1 -> Real-Imag to Complex/1
  GainH/1 -> Out1/1
  Gain/1 -> Sum1/2
  Delay/1 -> Gain/1
  Sum1/1 -> Delay/1, GainH/1

== system Filter_testaus_uusi/Highpass/HighpassH/Resonator157 ==
  In1 : Inport
  Constant : Constant  Value=0i
  Delay : Delay  DelayLength=1
  Gain : Gain  Gain=0.36657-0.93039i
  GainH : Gain  Gain=0.81871-0.57421i
  Real-Imag to Complex : RealImagToComplex
  Sum1 : Sum  Inputs=|++
  Out1 : Outport
  wires:
  Constant/1 -> Real-Imag to Complex/2
  Real-Imag to Complex/1 -> Sum1/1
  In1/1 -> Real-Imag to Complex/1
  GainH/1 -> Out1/1
  Gain/1 -> Sum1/2
  Delay/1 -> Gain/1
  Sum1/1 -> Delay/1, GainH/1

== system Filter_testaus_uusi/Highpass/HighpassH/Resonator158 ==
  In1 : Inport
  Constant : Constant  Value=0i
  Delay : Delay  DelayLength=1
  Gain : Gain  Gain=0.39229-0.91984i
  GainH : Gain  Gain=-0.82661+0.56277i
  Real-Imag to Complex : RealImagToComplex
  Sum1 : Sum  Inputs=|++
  Out1 : Outport
  wires:
  Constant/1 -> Real-Imag to Complex/2
  Real-Imag to Complex/1 -> Sum1/1
  In1/1 -> Real-Imag to Complex/1
  GainH/1 -> Out1/1
  Gain/1 -> Sum1/2
  Delay/1 -> Gain/1
  Sum1/1 -> Delay/1, GainH/1

== system Filter_testaus_uusi/Highpass/HighpassH/Resonator159 ==
  In1 : Inport
  Constant : Constant  Value=0i
  Delay : Delay  DelayLength=1
  Gain : Gain  Gain=0.41771-0.90858i
  GainH : Gain  Gain=0.83435-0.55123i
  Real-Imag to Complex : RealImagToComplex
  Sum1 : Sum  Inputs=|++
  Out1 : Outport
  wires:
  Constant/1 -> Real-Imag to Complex/2
  Real-Imag to Complex/1 -> Sum1/1
  In1/1 -> Real-Imag to Complex/1
  GainH/1 -> Out1/1
  Gain/1 -> Sum1/2
  Delay/1 -> Gain/1
  Sum1/1 -> Delay/1, GainH/1

== system Filter_testaus_uusi/Highpass/HighpassH/Resonator16 ==
  In1 : Inport
  Constant : Constant  Value=0i
  Delay : Delay  DelayLength=1
  Gain : Gain  Gain=0.39229+0.91984i
  GainH : Gain  Gain=-0.84194-0.53958i
  Real-Imag to Complex : RealImagToComplex
  Sum1 : Sum  Inputs=|++
  Out1 : Outport
  wires:
  Constant/1 -> Real-Imag to Complex/2
  Real-Imag to Complex/1 -> Sum1/1
  In1/1 -> Real-Imag to Complex/1
  GainH/1 -> Out1/1
  Gain/1 -> Sum1/2
  Delay/1 -> Gain/1
  Sum1/1 -> Delay/1, GainH/1

== system Filter_testaus_uusi/Highpass/HighpassH/Resonator160 ==
  In1 : Inport
  Constant : Constant  Value=0i
  Delay : Delay  DelayLength=1
  Gain : Gain  Gain=0.44281-0.89662i
  GainH : Gain  Gain=-0.84194+0.53958i
  Real-Imag to Complex : RealImagToComplex
  Sum1 : Sum  Inputs=|++
  Out1 : Outport
  wires:
  Constant/1 -> Real-Imag to Complex/2
  Real-Imag to Complex/1 -> Sum1/1
  In1/1 -> Real-Imag to Complex/1
  GainH/1 -> Out1/1
  Gain/1 -> Sum1/2
  Delay/1 -> Gain/1
  Sum1/1 -> Delay/1, GainH/1

== system Filter_testaus_uusi/Highpass/HighpassH/Resonator161 ==
  In1 : Inport
  Constant : Constant  Value=0i
  Delay : Delay  DelayLength=1
  Gain : Gain  Gain=0.46756-0.88396i
  GainH : Gain  Gain=0.84936-0.52782i
  Real-Imag to Complex : RealImagToComplex
  Sum1 : Sum  Inputs=|++
  Out1 : Outport
  wires:
  Constant/1 -> Real-Imag to Complex/2
  Real-Imag to Complex/1 -> Sum1/1
  In1/1 -> Real-Imag to Complex/1
  GainH/1 -> Out1/1
  Gain/1 -> Sum1/2
  Delay/1 -> Gain/1
  Sum1/1 -> Delay/1, GainH/1

== system Filter_testaus_uusi/Highpass/HighpassH/Resonator162 ==
  In1 : Inport
  Constant : Constant  Value=0i
  Delay : Delay  DelayLength=1
  Gain : Gain  Gain=0.49195-0.87062i
  GainH : Gain  Gain=-0.85661+0.51596i
  Real-Imag to Complex : RealImagToComplex
  Sum1 : Sum  Inputs=|++
  Out1 : Outport
  wires:
  Constant/1 -> Real-Imag to Complex/2
  Real-Imag to Complex/1 -> Sum1/1
  In1/1 -> Real-Imag to Complex/1
  GainH/1 -> Out1/1
  Gain/1 -> Sum1/2
  Delay/1 -> Gain/1
  Sum1/1 -> Delay/1, GainH/1

== system Filter_testaus_uusi/Highpass/HighpassH/Resonator163 ==
  In1 : Inport
  Constant : Constant  Value=0i
  Delay : Delay  DelayLength=1
  Gain : Gain  Gain=0.51596-0.85661i
  GainH : Gain  Gain=0.8637-0.50401i
  Real-Imag to Complex : RealImagToComplex
  Sum1 : Sum  Inputs=|++
  Out1 : Outport
  wires:
  Constant/1 -> Real-Imag to Complex/2
  Real-Imag to Complex/1 -> Sum1/1
  In1/1 -> Real-Imag to Complex/1
  GainH/1 -> Out1/1
  Gain/1 -> Sum1/2
  Delay/1 -> Gain/1
  Sum1/1 -> Delay/1, GainH/1

== system Filter_testaus_uusi/Highpass/HighpassH/Resonator164 ==
  In1 : Inport
  Constant : Constant  Value=0i
  Delay : Delay  DelayLength=1
  Gain : Gain  Gain=0.53958-0.84194i
  GainH : Gain  Gain=-0.87062+0.49195i
  Real-Imag to Complex : RealImagToComplex
  Sum1 : Sum  Inputs=|++
  Out1 : Outport
  wires:
  Constant/1 -> Real-Imag to Complex/2
  Real-Imag to Complex/1 -> Sum1/1
  In1/1 -> Real-Imag to Complex/1
  GainH/1 -> Out1/1
  Gain/1 -> Sum1/2
  Delay/1 -> Gain/1
  Sum1/1 -> Delay/1, GainH/1

== system Filter_testaus_uusi/Highpass/HighpassH/Resonator165 ==
  In1 : Inport
  Constant : Constant  Value=0i
  Delay : Delay  DelayLength=1
  Gain : Gain  Gain=0.56277-0.82661i
  GainH : Gain  Gain=0.87738-0.4798i
  Real-Imag to Complex : RealImagToComplex
  Sum1 : Sum  Inputs=|++
  Out1 : Outport
  wires:
  Constant/1 -> Real-Imag to Complex/2
  Real-Imag to Complex/1 -> Sum1/1
  In1/1 -> Real-Imag to Complex/1
  GainH/1 -> Out1/1
  Gain/1 -> Sum1/2
  Delay/1 -> Gain/1
  Sum1/1 -> Delay/1, GainH/1

== system Filter_testaus_uusi/Highpass/HighpassH/Resonator166 ==
  In1 : Inport
  Constant : Constant  Value=0i
  Delay : Delay  DelayLength=1
  Gain : Gain  Gain=0.58553-0.81065i
  GainH : Gain  Gain=-0.88396+0.46756i
  Real-Imag to Complex : RealImagToComplex
  Sum1 : Sum  Inputs=|++
  Out1 : Outport
  wires:
  Constant/1 -> Real-Imag to Complex/2
  Real-Imag to Complex/1 -> Sum1/1
  In1/1 -> Real-Imag to Complex/1
  GainH/1 -> Out1/1
  Gain/1 -> Sum1/2
  Delay/1 -> Gain/1
  Sum1/1 -> Delay/1, GainH/1

== system Filter_testaus_uusi/Highpass/HighpassH/Resonator167 ==
  In1 : Inport
  Constant : Constant  Value=0i
  Delay : Delay  DelayLength=1
  Gain : Gain  Gain=0.60784-0.79406i
  GainH : Gain  Gain=0.89037-0.45523i
  Real-Imag to Complex : RealImagToComplex
  Sum1 : Sum  Inputs=|++
  Out1 : Outport
  wires:
  Constant/1 -> Real-Imag to Complex/2
  Real-Imag to Complex/1 -> Sum1/1
  In1/1 -> Real-Imag to Complex/1
  GainH/1 -> Out1/1
  Gain/1 -> Sum1/2
  Delay/1 -> Gain/1
  Sum1/1 -> Delay/1, GainH/1

== system Filter_testaus_uusi/Highpass/HighpassH/Resonator168 ==
  In1 : Inport
  Constant : Constant  Value=0i
  Delay : Delay  DelayLength=1
  Gain : Gain  Gain=0.62968-0.77685i
  GainH : Gain  Gain=-0.89662+0.44281i
  Real-Imag to Complex : RealImagToComplex
  Sum1 : Sum  Inputs=|++
  Out1 : Outport
  wires:
  Constant/1 -> Real-Imag to Complex/2
  Real-Imag to Complex/1 -> Sum1/1
  In1/1 -> Real-Imag to Complex/1
  GainH/1 -> Out1/1
  Gain/1 -> Sum1/2
  Delay/1 -> Gain/1
  Sum1/1 -> Delay/1, GainH/1

== system Filter_testaus_uusi/Highpass/HighpassH/Resonator169 ==
  In1 : Inport
  Constant : Constant  Value=0i
  Delay : Delay  DelayLength=1
  Gain : Gain  Gain=0.65103-0.75905i
  GainH : Gain  Gain=0.90269-0.4303i
  Real-Imag to Complex : RealImagToComplex
  Sum1 : Sum  Inputs=|++
  Out1 : Outport
  wires:
  Constant/1 -> Real-Imag to Complex/2
  Real-Imag to Complex/1 -> Sum1/1
  In1/1 -> Real-Imag to Complex/1
  GainH/1 -> Out1/1
  Gain/1 -> Sum1/2
  Delay/1 -> Gain/1
  Sum1/1 -> Delay/1, GainH/1

== system Filter_testaus_uusi/Highpass/HighpassH/Resonator17 ==
  In1 : Inport
  Constant : Constant  Value=0i
  Delay : Delay  DelayLength=1
  Gain : Gain  Gain=0.36657+0.93039i
  GainH : Gain  Gain=0.83435+0.55123i
  Real-Imag to Complex : RealImagToComplex
  Sum1 : Sum  Inputs=|++
  Out1 : Outport
  wires:
  Constant/1 -> Real-Imag to Complex/2
  Real-Imag to Complex/1 -> Sum1/1
  In1/1 -> Real-Imag to Complex/1
  GainH/1 -> Out1/1
  Gain/1 -> Sum1/2
  Delay/1 -> Gain/1
  Sum1/1 -> Delay/1, GainH/1

== system Filter_testaus_uusi/Highpass/HighpassH/Resonator170 ==
  In1 : Inport
  Constant : Constant  Value=0i
  Delay : Delay  DelayLength=1
  Gain : Gain  Gain=0.67188-0.74066i
  GainH : Gain  Gain=-0.90858+0.41771i
  Real-Imag to Complex : RealImagToComplex
  Sum1 : Sum  Inputs=|++
  Out1 : Outport
  wires:
  Constant/1 -> Real-Imag to Complex/2
  Real-Imag to Complex/1 -> Sum1/1
  In1/1 -> Real-Imag to Complex/1
  GainH/1 -> Out1/1
  Gain/1 -> Sum1/2
  Delay/1 -> Gain/1
  Sum1/1 -> Delay/1, GainH/1

== system Filter_testaus_uusi/Highpass/HighpassH/Resonator171 ==
  In1 : Inport
  Constant : Constant  Value=0i
  Delay : Delay  DelayLength=1
  Gain : Gain  Gain=0.69221-0.7217i
  GainH : Gain  Gain=0.9143-0.40504i
  Real-Imag to Complex : RealImagToComplex
  Sum1 : Sum  Inputs=|++
  Out1 : Outport
  wires:
  Constant/1 -> Real-Imag to Complex/2
  Real-Imag to Complex/1 -> Sum1/1
  In1/1 -> Real-Imag to Complex/1
  GainH/1 -> Out1/1
  Gain/1 -> Sum1/2
  Delay/1 -> Gain/1
  Sum1/1 -> Delay/1, GainH/1

== system Filter_testaus_uusi/Highpass/HighpassH/Resonator172 ==
  In1 : Inport
  Constant : Constant  Value=0i
  Delay : Delay  DelayLength=1
  Gain : Gain  Gain=0.712-0.70218i
  GainH : Gain  Gain=-0.91984+0.39229i
  Real-Imag to Complex : RealImagToComplex
  Sum1 : Sum  Inputs=|++
  Out1 : Outport
  wires:
  Constant/1 -> Real-Imag to Complex/2
  Real-Imag to Complex/1 -> Sum1/1
  In1/1 -> Real-Imag to Complex/1
  GainH/1 -> Out1/1
  Gain/1 -> Sum1/2
  Delay/1 -> Gain/1
  Sum1/1 -> Delay/1, GainH/1

== system Filter_testaus_uusi/Highpass/HighpassH/Resonator173 ==
  In1 : Inport
  Constant : Constant  Value=0i
  Delay : Delay  DelayLength=1
  Gain : Gain  Gain=0.73125-0.68211i
  GainH : Gain  Gain=0.9252-0.37947i
  Real-Imag to Complex : RealImagToComplex
  Sum1 : Sum  Inputs=|++
  Out1 : Outport
  wires:
  Constant/1 -> Real-Imag to Complex/2
  Real-Imag to Complex/1 -> Sum1/1
  In1/1 -> Real-Imag to Complex/1
  GainH/1 -> Out1/1
  Gain/1 -> Sum1/2
  Delay/1 -> Gain/1
  Sum1/1 -> Delay/1, GainH/1

== system Filter_testaus_uusi/Highpass/HighpassH/Resonator174 ==
  In1 : Inport
  Constant : Constant  Value=0i
  Delay : Delay  DelayLength=1
  Gain : Gain  Gain=0.74993-0.66152i
  GainH : Gain  Gain=-0.93039+0.36657i
  Real-Imag to Complex : RealImagToComplex
  Sum1 : Sum  Inputs=|++
  Out1 : Outport
  wires:
  Constant/1 -> Real-Imag to Complex/2
  Real-Imag to Complex/1 -> Sum1/1
  In1/1 -> Real-Imag to Complex/1
  GainH/1 -> Out1/1
  Gain/1 -> Sum1/2
  Delay/1 -> Gain/1
  Sum1/1 -> Delay/1, GainH/1

== system Filter_testaus_uusi/Highpass/HighpassH/Resonator175 ==
  In1 : Inport
  Constant : Constant  Value=0i
  Delay : Delay  DelayLength=1
  Gain : Gain  Gain=0.76803-0.64042i
  GainH : Gain  Gain=0.93539-0.3536i
  Real-Imag to Complex : RealImagToComplex
  Sum1 : Sum  Inputs=|++
  Out1 : Outport
  wires:
  Constant/1 -> Real-Imag to Complex/2
  Real-Imag to Complex/1 -> Sum1/1
  In1/1 -> Real-Imag to Complex/1
  GainH/1 -> Out1/1
  Gain/1 -> Sum1/2
  Delay/1 -> Gain/1
  Sum1/1 -> Delay/1, GainH/1

== system Filter_testaus_uusi/Highpass/HighpassH/Resonator18 ==
  In1 : Inport
  Constant : Constant  Value=0i
  Delay : Delay  DelayLength=1
  Gain : Gain  Gain=0.34057+0.94022i
  GainH : Gain  Gain=-0.82661-0.56277i
  Real-Imag to Complex : RealImagToComplex
  Sum1 : Sum  Inputs=|++
  Out1 : Outport
  wires:
  Constant/1 -> Real-Imag to Complex/2
  Real-Imag to Complex/1 -> Sum1/1
  In1/1 -> Real-Imag to Complex/1
  GainH/1 -> Out1/1
  Gain/1 -> Sum1/2
  Delay/1 -> Gain/1
  Sum1/1 -> Delay/1, GainH/1

== system Filter_testaus_uusi/Highpass/HighpassH/Resonator19 ==
  In1 : Inport
  Constant : Constant  Value=0i
  Delay : Delay  DelayLength=1
  Gain : Gain  Gain=0.3143+0.94932i
  GainH : Gain  Gain=0.81871+0.57421i
  Real-Imag to Complex : RealImagToComplex
  Sum1 : Sum  Inputs=|++
  Out1 : Outport
  wires:
  Constant/1 -> Real-Imag to Complex/2
  Real-Imag to Complex/1 -> Sum1/1
  In1/1 -> Real-Imag to Complex/1
  GainH/1 -> Out1/1
  Gain/1 -> Sum1/2
  Delay/1 -> Gain/1
  Sum1/1 -> Delay/1, GainH/1

== system Filter_testaus_uusi/Highpass/HighpassH/Resonator2 ==
  In1 : Inport
  Constant : Constant  Value=0i
  Delay : Delay  DelayLength=1
  Gain : Gain  Gain=0.712+0.70218i
  GainH : Gain  Gain=-0.93039-0.36657i
  Real-Imag to Complex : RealImagToComplex
  Sum1 : Sum  Inputs=|++
  Out1 : Outport
  wires:
  Constant/1 -> Real-Imag to Complex/2
  Real-Imag to Complex/1 -> Sum1/1
  In1/1 -> Real-Imag to Complex/1
  GainH/1 -> Out1/1
  Gain/1 -> Sum1/2
  Delay/1 -> Gain/1
  Sum1/1 -> Delay/1, GainH/1

== system Filter_testaus_uusi/Highpass/HighpassH/Resonator20 ==
  In1 : Inport
  Constant : Constant  Value=0i
  Delay : Delay  DelayLength=1
  Gain : Gain  Gain=0.28779+0.95769i
  GainH : Gain  Gain=-0.81065-0.58553i
  Real-Imag to Complex : RealImagToComplex
  Sum1 : Sum  Inputs=|++
  Out1 : Outport
  wires:
  Constant/1 -> Real-Imag to Complex/2
  Real-Imag to Complex/1 -> Sum1/1
  In1/1 -> Real-Imag to Complex/1
  GainH/1 -> Out1/1
  Gain/1 -> Sum1/2
  Delay/1 -> Gain/1
  Sum1/1 -> Delay/1, GainH/1

== system Filter_testaus_uusi/Highpass/HighpassH/Resonator21 ==
  In1 : Inport
  Constant : Constant  Value=0i
  Delay : Delay  DelayLength=1
  Gain : Gain  Gain=0.26106+0.96532i
  GainH : Gain  Gain=0.80243+0.59675i
  Real-Imag to Complex : RealImagToComplex
  Sum1 : Sum  Inputs=|++
  Out1 : Outport
  wires:
  Constant/1 -> Real-Imag to Complex/2
  Real-Imag to Complex/1 -> Sum1/1
  In1/1 -> Real-Imag to Complex/1
  GainH/1 -> Out1/1
  Gain/1 -> Sum1/2
  Delay/1 -> Gain/1
  Sum1/1 -> Delay/1, GainH/1

== system Filter_testaus_uusi/Highpass/HighpassH/Resonator22 ==
  In1 : Inport
  Constant : Constant  Value=0i
  Delay : Delay  DelayLength=1
  Gain : Gain  Gain=0.23412+0.97221i
  GainH : Gain  Gain=-0.79406-0.60784i
  Real-Imag to Complex : RealImagToComplex
  Sum1 : Sum  Inputs=|++
  Out1 : Outport
  wires:
  Constant/1 -> Real-Imag to Complex/2
  Real-Imag to Complex/1 -> Sum1/1
  In1/1 -> Real-Imag to Complex/1
  GainH/1 -> Out1/1
  Gain/1 -> Sum1/2
  Delay/1 -> Gain/1
  Sum1/1 -> Delay/1, GainH/1

== system Filter_testaus_uusi/Highpass/HighpassH/Resonator23 ==
  In1 : Inport
  Constant : Constant  Value=0i
  Delay : Delay  DelayLength=1
  Gain : Gain  Gain=0.20701+0.97834i
  GainH : Gain  Gain=0.78553+0.61882i
  Real-Imag to Complex : RealImagToComplex
  Sum1 : Sum  Inputs=|++
  Out1 : Outport
  wires:
  Constant/1 -> Real-Imag to Complex/2
  Real-Imag to Complex/1 -> Sum1/1
  In1/1 -> Real-Imag to Complex/1
  GainH/1 -> Out1/1
  Gain/1 -> Sum1/2
  Delay/1 -> Gain/1
  Sum1/1 -> Delay/1, GainH/1

== system Filter_testaus_uusi/Highpass/HighpassH/Resonator24 ==
  In1 : Inport
  Constant : Constant  Value=0i
  Delay : Delay  DelayLength=1
  Gain : Gain  Gain=0.17973+0.98372i
  GainH : Gain  Gain=-0.77685-0.62968i
  Real-Imag to Complex : RealImagToComplex
  Sum1 : Sum  Inputs=|++
  Out1 : Outport
  wires:
  Constant/1 -> Real-Imag to Complex/2
  Real-Imag to Complex/1 -> Sum1/1
  In1/1 -> Real-Imag to Complex/1
  GainH/1 -> Out1/1
  Gain/1 -> Sum1/2
  Delay/1 -> Gain/1
  Sum1/1 -> Delay/1, GainH/1

== system Filter_testaus_uusi/Highpass/HighpassH/Resonator25 ==
  In1 : Inport
  Constant : Constant  Value=0i
  Delay : Delay  DelayLength=1
  Gain : Gain  Gain=0.15231+0.98833i
  GainH : Gain  Gain=0.76803+0.64042i
  Real-Imag to Complex : RealImagToComplex
  Sum1 : Sum  Inputs=|++
  Out1 : Outport
  wires:
  Constant/1 -> Real-Imag to Complex/2
  Real-Imag to Complex/1 -> Sum1/1
  In1/1 -> Real-Imag to Complex/1
  GainH/1 -> Out1/1
  Gain/1 -> Sum1/2
  Delay/1 -> Gain/1
  Sum1/1 -> Delay/1, GainH/1

== system Filter_testaus_uusi/Highpass/HighpassH/Resonator26 ==
  In1 : Inport
  Constant : Constant  Value=0i
  Delay : Delay  DelayLength=1
  Gain : Gain  Gain=0.12478+0.99218i
  GainH : Gain  Gain=-0.75905-0.65103i
  Real-Imag to Complex : RealImagToComplex
  Sum1 : Sum  Inputs=|++
  Out1 : Outport
  wires:
  Constant/1 -> Real-Imag to Complex/2
  Real-Imag to Complex/1 -> Sum1/1
  In1/1 -> Real-Imag to Complex/1
  GainH/1 -> Out1/1
  Gain/1 -> Sum1/2
  Delay/1 -> Gain/1
  Sum1/1 -> Delay/1, GainH/1

== system Filter_testaus_uusi/Highpass/HighpassH/Resonator27 ==
  In1 : Inport
  Constant : Constant  Value=0i
  Delay : Delay  DelayLength=1
  Gain : Gain  Gain=0.097152+0.99527i
  GainH : Gain  Gain=0.74993+0.66152i
  Real-Imag to Complex : RealImagToComplex
  Sum1 : Sum  Inputs=|++
  Out1 : Outport
  wires:
  Constant/1 -> Real-Imag to Complex/2
  Real-Imag to Complex/1 -> Sum1/1
  In1/1 -> Real-Imag to Complex/1
  GainH/1 -> Out1/1
  Gain/1 -> Sum1/2
  Delay/1 -> Gain/1
  Sum1/1 -> Delay/1, GainH/1

== system Filter_testaus_uusi/Highpass/HighpassH/Resonator28 ==
  In1 : Inport
  Constant : Constant  Value=0i
  Delay : Delay  DelayLength=1
  Gain : Gain  Gain=0.069448+0.99759i
  GainH : Gain  Gain=-0.74066-0.67188i
  Real-Imag to Complex : RealImagToComplex
  Sum1 : Sum  Inputs=|++
  Out1 : Outport
  wires:
  Constant/1 -> Real-Imag to Complex/2
  Real-Imag to Complex/1 -> Sum1/1
  In1/1 -> Real-Imag to Complex/1
  GainH/1 -> Out1/1
  Gain/1 -> Sum1/2
  Delay/1 -> Gain/1
  Sum1/1 -> Delay/1, GainH/1

== system Filter_testaus_uusi/Highpass/HighpassH/Resonator29 ==
  In1 : Inport
  Constant : Constant  Value=0i
  Delay : Delay  DelayLength=1
  Gain : Gain  Gain=0.04169+0.99913i
  GainH : Gain  Gain=0.73125+0.68211i
  Real-Imag to Complex : RealImagToComplex
  Sum1 : Sum  Inputs=|++
  Out1 : Outport
  wires:
  Constant/1 -> Real-Imag to Complex/2
  Real-Imag to Complex/1 -> Sum1/1
  In1/1 -> Real-Imag to Complex/1
  GainH/1 -> Out1/1
  Gain/1 -> Sum1/2
  Delay/1 -> Gain/1
  Sum1/1 -> Delay/1, GainH/1

== system Filter_testaus_uusi/Highpass/HighpassH/Resonator3 ==
  In1 : Inport
  Constant : Constant  Value=0i
  Delay : Delay  DelayLength=1
  Gain : Gain  Gain=0.69221+0.7217i
  GainH : Gain  Gain=0.9252+0.37947i
  Real-Imag to Complex : RealImagToComplex
  Sum1 : Sum  Inputs=|++
  Out1 : Outport
  wires:
  Constant/1 -> Real-Imag to Complex/2
  Real-Imag to Complex/1 -> Sum1/1
  In1/1 -> Real-Imag to Complex/1
  GainH/1 -> Out1/1
  Gain/1 -> Sum1/2
  Delay/1 -> Gain/1
  Sum1/1 -> Delay/1, GainH/1
